simulink model "inputValidation"  (R2022b)
settings: Solver=ode45  StartTime=0.0  StopTime=10.0  RelTol=1e-3  EnableMultiTasking=on
PreLoadFcn:
  | load allParamValues.mat
undefined symbols (not defined in the file or in its folder): J, Ki, Km, Kp, Ts
libraries: simulink x1, SignalEditorBlockLib x1
settings Model: Creator=jrivitus  LastModifiedBy=bensweet
settings SolverCC: MaxConsecutiveZCs=25  AlgebraicLoopSolver=TrustRegion  MaxZcPerStep=1
settings DataIOCC: LimitDataPoints=on  SaveFormat=Array  ReturnWorkspaceOutputs=off
settings OptimizationCC: ExpressionDepthLimit=2147483647  InitFltsAndDblsToZero=on  LifeSpan=inf
settings DebuggingCC: UnconnectedInputMsg=warning  UnconnectedOutputMsg=warning  UnconnectedLineMsg=warning  PregeneratedLibrarySubsystemCodeDiagnostic=none  SFMachineParentedDataDiag=warning
settings HardwareCC: ProdBitPerPointer=32  ProdBitPerSizeT=32  ProdBitPerPtrDiffT=32  ProdLargestAtomicFloat=None  ProdIntDivRoundTo=Undefined  ProdEndianess=Unspecified  ProdWordSize=32  ProdHWDeviceType=32-bit Generic
settings ModelReferenceCC: EnableRefExpFcnMdlSchedulingChecks=on  PropagateSignalLabelsOutOfModel=off
settings SFSimCC: SimUseLocalCustomCode=off
settings RTWCC: RTWUseLocalCustomCode=off  DLArmComputeVersion=19.05
settings CodeAppCC: StateflowObjectComments=on
settings GRTTargetCC: TargetLangStandard=C89/C90 (ANSI)  CombineOutputUpdateFcns=off  GRTInterface=on
settings ConfigComp: CovMetricSettings=dw  CovSaveCumulativeToWorkspaceVar=on  CovSaveSingleToWorkspaceVar=on  CovExternalEMLEnable=off  CovSFcnEnable=off

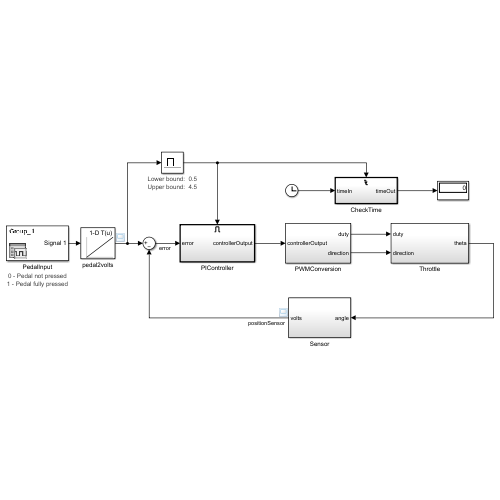
[thumbnail: Simulink's stored preview of the top-level diagram]
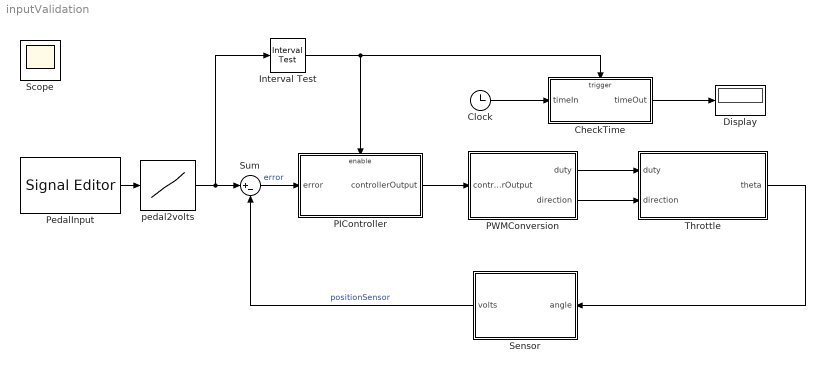
== system inputValidation ==
  CheckTime : Subsystem  TreatAsAtomicUnit=on
  Clock : Clock
  Display : Display
  Interval Test : simulink/Logic and Bit Operations/Interval Test  IntervalClosedRight=on  uplimit=4.5  IntervalClosedLeft=on  lowlimit=0.5  OutDataTypeStr=boolean
      settings: AttributesFormatString="Lower bound:  %<lowlimit>\\nUpper bound:  %<uplimit>"
  PIController : Subsystem
  PWMConversion : Subsystem
  PedalInput : SignalEditorBlockLib/Signal Editor  FileName=PedalInput_dataset.mat  ActiveScenario=Group_1  ActiveSignal=Signal 1  IsBus=off  OutputBusObjectStr=Bus: BusObject  SampleTime=0  OutputAfterFinalValue=Extrapolation  Unit=inherit  PreserveSignalName=on
      settings: AttributesFormatString=0 - Pedal not pressed\n1 - Pedal fully pressed
  Sensor : Subsystem
  Sum : Sum  Inputs=|+-
  Throttle : Subsystem
  pedal2volts : Lookup_n-D  NumberOfTableDimensions=1  BreakpointsForDimension1=[0 1]  Table=[0.5 4.5]  RndMeth=Simplest
  Scope : Scope
  wires:
  pedal2volts/1 -> Sum/1, Interval Test/1
  Sum/1 -> PIController/1(error)  "error"
  PIController/1(controllerOutput) -> PWMConversion/1(controllerOutput)
  PWMConversion/1(duty) -> Throttle/1(duty)
  PWMConversion/2(direction) -> Throttle/2(direction)
  Sensor/1(volts) -> Sum/2  "positionSensor"
  Throttle/1(theta) -> Sensor/1(angle)
  PedalInput/1 -> pedal2volts/1
  Interval Test/1 -> PIController/Enable, CheckTime/Trigger
  Clock/1 -> CheckTime/1(timeIn)
  CheckTime/1(timeOut) -> Display/1

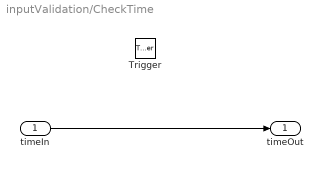
== system inputValidation/CheckTime ==
  timeIn : Inport
  Trigger : TriggerPort  TriggerType=falling  VariantControl=Variant
  timeOut : Outport  VectorParamsAs1DForOutWhenUnconnected=off
  wires:
  timeIn/1 -> timeOut/1

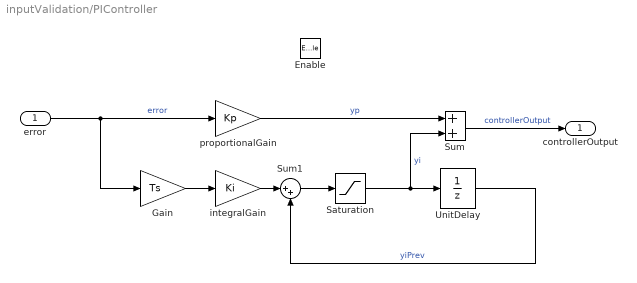
== system inputValidation/PIController ==
  error : Inport
  Enable : EnablePort
  Gain : Gain  Gain=Ts  SaturateOnIntegerOverflow=on  OutDataTypeStr=Inherit: Same as input  ParamDataTypeStr=Inherit: Same as input
  Saturation : Saturate  UpperLimit=1  LowerLimit=-1
      settings: AttributesFormatString=Max: %<UpperLimit>\nMin: %<LowerLimit>
  Sum : Sum  InputSameDT=on  SaturateOnIntegerOverflow=on  OutDataTypeStr=Inherit: Same as first input
  Sum1 : Sum  Inputs=|++  InputSameDT=on  SaturateOnIntegerOverflow=on  OutDataTypeStr=Inherit: Same as first input
  UnitDelay : UnitDelay  SampleTime=Ts  HasFrameUpgradeWarning=on
      settings: AttributesFormatString=yi0 = %<X0>\nSample time = %<SampleTime>
  integralGain : Gain  Gain=Ki  SaturateOnIntegerOverflow=on  OutDataTypeStr=Inherit: Same as input  ParamDataTypeStr=Inherit: Same as input
  proportionalGain : Gain  Gain=Kp  SaturateOnIntegerOverflow=on  OutDataTypeStr=Inherit: Same as input  ParamDataTypeStr=Inherit: Same as input
  controllerOutput : Outport  VectorParamsAs1DForOutWhenUnconnected=off
  wires:
  Sum/1 -> controllerOutput/1  "controllerOutput"
  Saturation/1 -> Sum/2, UnitDelay/1  "yi"
  Sum1/1 -> Saturation/1
  UnitDelay/1 -> Sum1/2  "yiPrev"
  Gain/1 -> integralGain/1
  integralGain/1 -> Sum1/1
  proportionalGain/1 -> Sum/1  "yp"
  error/1 -> proportionalGain/1, Gain/1  "error"

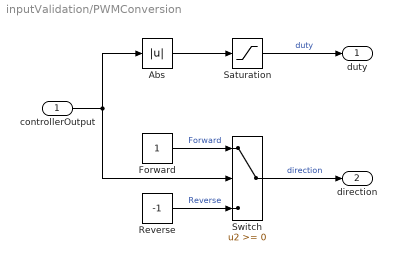
== system inputValidation/PWMConversion ==
  controllerOutput : Inport
  Abs : Abs  SaturateOnIntegerOverflow=off
  Forward : Constant  OutDataTypeStr=double
  Reverse : Constant  Value=-1  OutDataTypeStr=double
  Saturation : Saturate  UpperLimit=1  LowerLimit=0
      settings: AttributesFormatString=%<LowerLimit> < duty < %<UpperLimit>
  Switch : Switch  SaturateOnIntegerOverflow=off  InputSameDT=off
      settings: AttributesFormatString=Criteria: %<Criteria>\nThreshold: %<Threshold>
  duty : Outport  VectorParamsAs1DForOutWhenUnconnected=off
  direction : Outport  Port=2  VectorParamsAs1DForOutWhenUnconnected=off
  wires:
  controllerOutput/1 -> Abs/1, Switch/2
  Forward/1 -> Switch/1  "Forward"
  Reverse/1 -> Switch/3  "Reverse"
  Switch/1 -> direction/1  "direction"
  Saturation/1 -> duty/1  "duty"
  Abs/1 -> Saturation/1

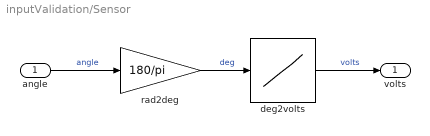
== system inputValidation/Sensor ==
  angle : Inport
  deg2volts : Lookup_n-D  NumberOfTableDimensions=1  BreakpointsForDimension1=[0 90]  Table=[0.5 4.5]  RndMeth=Simplest
  rad2deg : Gain  Gain=180/pi  SaturateOnIntegerOverflow=on  OutDataTypeStr=Inherit: Same as input  ParamDataTypeStr=Inherit: Same as input
  volts : Outport  VectorParamsAs1DForOutWhenUnconnected=off
  wires:
  rad2deg/1 -> deg2volts/1  "deg"
  deg2volts/1 -> volts/1  "volts"
  angle/1 -> rad2deg/1  "angle"

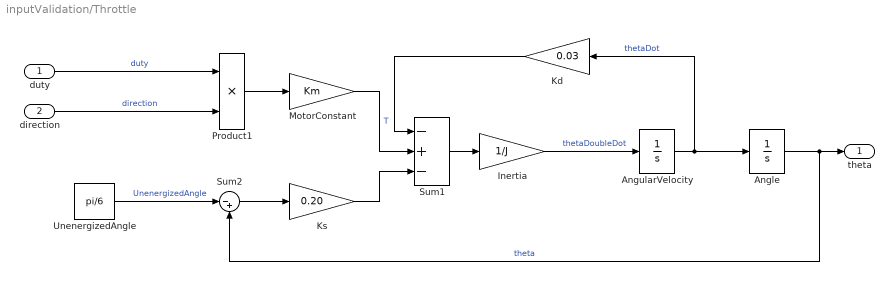
== system inputValidation/Throttle ==
  duty : Inport
  direction : Inport  Port=2
  Angle : Integrator  InitialCondition=pi/6  LimitOutput=on  UpperSaturationLimit=pi/2  LowerSaturationLimit=0
      settings: AttributesFormatString=Initial condition: %<InitialCondition>\n%<LowerSaturationLimit> <= theta <= %<UpperSaturationLimit>
  AngularVelocity : Integrator
      settings: AttributesFormatString=Initial condition: %<InitialCondition>
  Inertia : Gain  Gain=1/J  SaturateOnIntegerOverflow=on  OutDataTypeStr=Inherit: Same as input  ParamDataTypeStr=Inherit: Same as input
  Kd : Gain  Gain=0.03  SaturateOnIntegerOverflow=on  OutDataTypeStr=Inherit: Same as input  ParamDataTypeStr=Inherit: Same as input
  Ks : Gain  Gain=0.20  SaturateOnIntegerOverflow=on  OutDataTypeStr=Inherit: Same as input  ParamDataTypeStr=Inherit: Same as input
  MotorConstant : Gain  Gain=Km  SaturateOnIntegerOverflow=on  OutDataTypeStr=Inherit: Same as input  ParamDataTypeStr=Inherit: Same as input
  Product1 : Product  SaturateOnIntegerOverflow=on  OutDataTypeStr=Inherit: Same as first input
  Sum1 : Sum  Inputs=-+-  SaturateOnIntegerOverflow=on
  Sum2 : Sum  Inputs=|-+  SaturateOnIntegerOverflow=on
  UnenergizedAngle : Constant  Value=pi/6
  theta : Outport  VectorParamsAs1DForOutWhenUnconnected=off
  wires:
  Ks/1 -> Sum1/3
  Kd/1 -> Sum1/1
  MotorConstant/1 -> Sum1/2  "T"
  duty/1 -> Product1/1  "duty"
  direction/1 -> Product1/2  "direction"
  Sum1/1 -> Inertia/1
  Inertia/1 -> AngularVelocity/1  "thetaDoubleDot"
  AngularVelocity/1 -> Kd/1, Angle/1  "thetaDot"
  Angle/1 -> Sum2/2, theta/1  "theta"
  Sum2/1 -> Ks/1
  UnenergizedAngle/1 -> Sum2/1  "UnenergizedAngle"
  Product1/1 -> MotorConstant/1
